simulink library "LPFilter"  (R2018b)
settings: Solver=VariableStepAuto  StartTime=0.0  StopTime=10.0  RelTol=1e-3
settings Model: Creator=linqi  LastModifiedBy=linqi

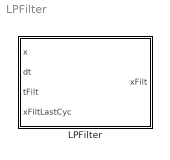
== system LPFilter ==
  LPFilter : Subsystem

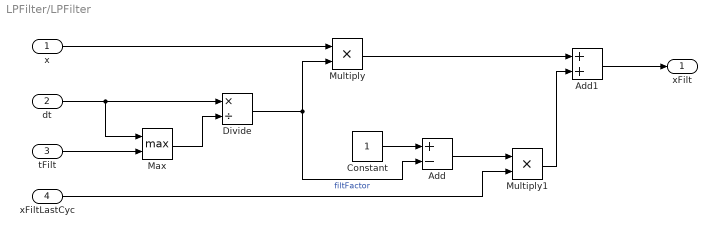
== system LPFilter/LPFilter ==
  x : Inport  OutDataTypeStr=single
  dt : Inport  Port=2  OutDataTypeStr=single
  tFilt : Inport  Port=3  OutDataTypeStr=single
  xFiltLastCyc : Inport  Port=4  OutDataTypeStr=single
  Add : Sum  Inputs=+-
  Add1 : Sum
  Constant : Constant  OutDataTypeStr=single
  Divide : Product  Inputs=*/
  Max : MinMax  Function=max  Inputs=2
  Multiply : Product
  Multiply1 : Product
  xFilt : Outport
  wires:
  Multiply/1 -> Add1/1
  Constant/1 -> Add/1
  dt/1 -> Divide/1, Max/1
  tFilt/1 -> Max/2
  Divide/1 -> Add/2, Multiply/2  "filtFactor"
  Add1/1 -> xFilt/1
  Add/1 -> Multiply1/1
  xFiltLastCyc/1 -> Multiply1/2
  Max/1 -> Divide/2
  Multiply1/1 -> Add1/2
  x/1 -> Multiply/1
